simulink model "LQI_2017a"  (R2017a)
settings: Solver=VariableStepAuto  StartTime=0.0  StopTime=4  RelTol=1e-3
values from neighbouring files (symbols this model uses):
  Cr = [0 0 1]    [ventilador.m]
  Klqi = lqi(sis,Q,R)    [ControladorMotor.m]    (also in ventilador.m = [Klqi Klqi(end)])
  L = P*C'*(1/R_L)    [ventilador.m]
  Ts = 0.01    [ventilador.m]
undefined symbols (not defined in the file or in its folder): A, B, C, D
settings Model: Creator=jacqu  LastModifiedBy=jacqu
settings SFSimCC: SimUseLocalCustomCode=on
settings RTWCC: RTWUseLocalCustomCode=on

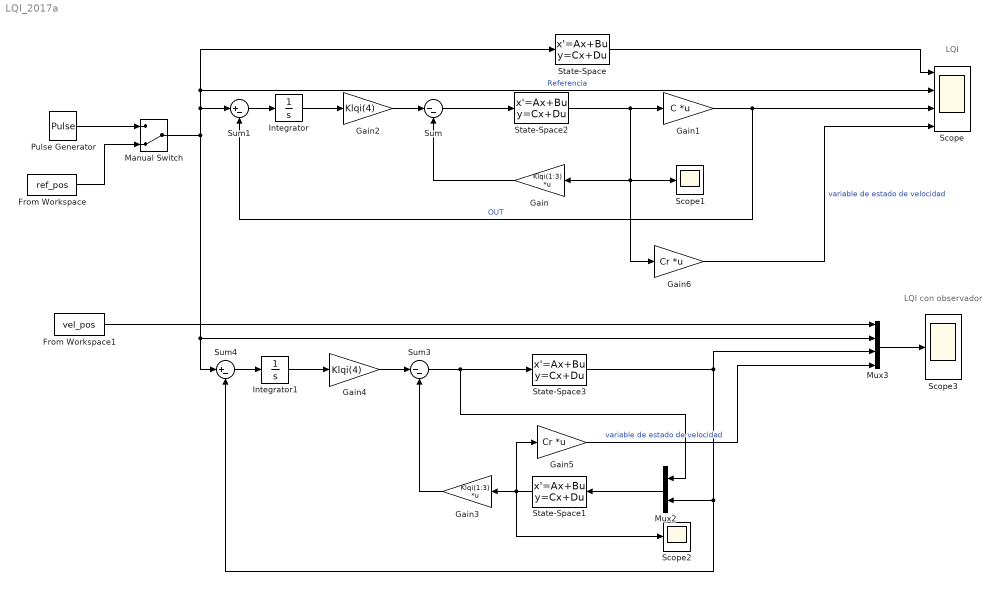
== system LQI_2017a ==
  note: LQI con observador
  note: LQI
  From Workspace : FromWorkspace  VariableName=ref_pos  SampleTime=Ts
  From Workspace1 : FromWorkspace  VariableName=vel_pos  SampleTime=Ts
  Gain : Gain  Gain=Klqi(1:3)  Multiplication=Matrix(K*u) (u vector)
  Gain1 : Gain  Gain=C  Multiplication=Matrix(K*u) (u vector)
  Gain2 : Gain  Gain=Klqi(4)
  Gain3 : Gain  Gain=Klqi(1:3)  Multiplication=Matrix(K*u) (u vector)
  Gain4 : Gain  Gain=Klqi(4)
  Gain5 : Gain  Gain=Cr  Multiplication=Matrix(K*u) (u vector)
  Gain6 : Gain  Gain=Cr  Multiplication=Matrix(K*u) (u vector)
  Integrator : Integrator
  Integrator1 : Integrator
  Manual Switch : ManualSwitch  CurrentSetting=0
  Mux2 : Mux  Inputs=2
  Mux3 : Mux
  Pulse Generator : DiscretePulseGenerator  PulseType=Time based  Period=1/0.5  PulseWidth=50
  Scope : Scope  NumInputPorts=4
  Scope1 : Scope
  Scope2 : Scope
  Scope3 : Scope
  State-Space : StateSpace  A=A  B=B  C=C  D=D  X0=0
  State-Space1 : StateSpace  A=A-L*C  B=[B L]  C=eye(3)  D=zeros(3,2)  X0=0
  State-Space2 : StateSpace  A=A  B=B  C=eye(3)  D=zeros(3,1)  X0=0
  State-Space3 : StateSpace  A=A  B=B  C=C  D=D  X0=0
  Sum : Sum  Inputs=|--
  Sum1 : Sum  Inputs=|+-
  Sum3 : Sum  Inputs=|--
  Sum4 : Sum  Inputs=|+-
  wires:
  Manual Switch/1 -> State-Space/1, Scope/2, Sum1/1, Mux3/2, Sum4/1  "Referencia"
  Gain/1 -> Sum/2
  State-Space/1 -> Scope/1
  Gain1/1 -> Scope/3, Sum1/2  "OUT"
  Sum/1 -> State-Space2/1
  State-Space2/1 -> Gain6/1, Gain/1, Scope1/1, Gain1/1
  Sum1/1 -> Integrator/1
  Integrator/1 -> Gain2/1
  Gain2/1 -> Sum/1
  Pulse Generator/1 -> Manual Switch/1
  From Workspace/1 -> Manual Switch/2
  State-Space1/1 -> Gain5/1, Scope2/1, Gain3/1
  Mux3/1 -> Scope3/1
  Gain3/1 -> Sum3/2
  Sum4/1 -> Integrator1/1
  Mux2/1 -> State-Space1/1
  State-Space3/1 -> Mux2/2, Sum4/2, Mux3/3
  Sum3/1 -> Mux2/1, State-Space3/1
  Gain4/1 -> Sum3/1
  Integrator1/1 -> Gain4/1
  Gain5/1 -> Mux3/4  "variable de estado de velocidad"
  From Workspace1/1 -> Mux3/1
  Gain6/1 -> Scope/4  "variable de estado de velocidad"
